simulink model "simulation_stoerung"  (Simulink 7.0)
settings: Solver=ode45  StartTime=0.0  StopTime=10  RelTol=1e-3
settings Model: Creator=Matze  LastModifiedBy=Matze

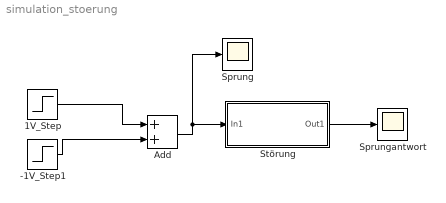
== system simulation_stoerung ==
  -1V_Step1 : Step  Time=5  After=-1  SampleTime=0
  1V_Step : Step  SampleTime=0
  Add : Sum  OutDataType=sfix(16)  OutScaling=2^-10
  Sprung : Scope
      settings: TimeRange=1  YMin=2.5  YMax=3.5  SaveName=ScopeOut  DataFormat=Array
  Sprungantwort : Scope
      settings: TimeRange=1  YMin=2.5  YMax=3.5  SaveName=ScopeOut1  DataFormat=Array
  Störung : Subsystem
  wires:
  1V_Step/1 -> Add/1
  Add/1 -> Störung/1(In1), Sprung/1
  Störung/1(Out1) -> Sprungantwort/1
  -1V_Step1/1 -> Add/2

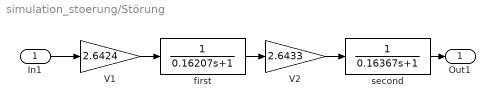
== system simulation_stoerung/Störung ==
  In1 : Inport  OutDataType=sfix(16)  OutScaling=2^0
  V1 : Gain  Gain=2.6424  ParameterDataType=sfix(16)  ParameterScaling=2^0  OutDataType=sfix(16)  OutScaling=2^0
  V2 : Gain  Gain=2.6433  ParameterDataType=sfix(16)  ParameterScaling=2^0  OutDataType=sfix(16)  OutScaling=2^0
  first : TransferFcn  Denominator=[0.16207 1]
  second : TransferFcn  Denominator=[0.16367 1]
  Out1 : Outport  OutDataType=sfix(16)  OutScaling=2^0
  wires:
  In1/1 -> V1/1
  V1/1 -> first/1
  first/1 -> V2/1
  second/1 -> Out1/1
  V2/1 -> second/1
